simulink model "systemlin"  (R2020b)
settings: Solver=VariableStepAuto  StartTime=0.0  StopTime=10.0  RelTol=1e-3
values from neighbouring files (symbols this model uses):
  a1 = -0.1    [PID_control.m]
  g = p(11,1)    [ModifiedFourTankSystem.m]    (also in approx_MPC_Soft_Output_Input_Constrained.m = [gu;zeros(length(gu),1)]; det_lin_MPC_Soft_Output_Input_Constrained.m = [gu;zeros(length(gu),1)]; noise_nonlin_MPC_Soft_Output_Input_Constrained.m = [gu;zeros(length(gu),1)]; nonlin_MPC_Soft_Output_Input_Constrained.m = [gu;zeros(length(gu),1)])
  rho = p(12,1)    [ModifiedFourTankSystem.m]
undefined symbols (not defined in the file or in its folder): A1, A2, a2, A3, a3, A4, a4, gam1, gam2
settings Model: Creator=maxfi  LastModifiedBy=maxfi

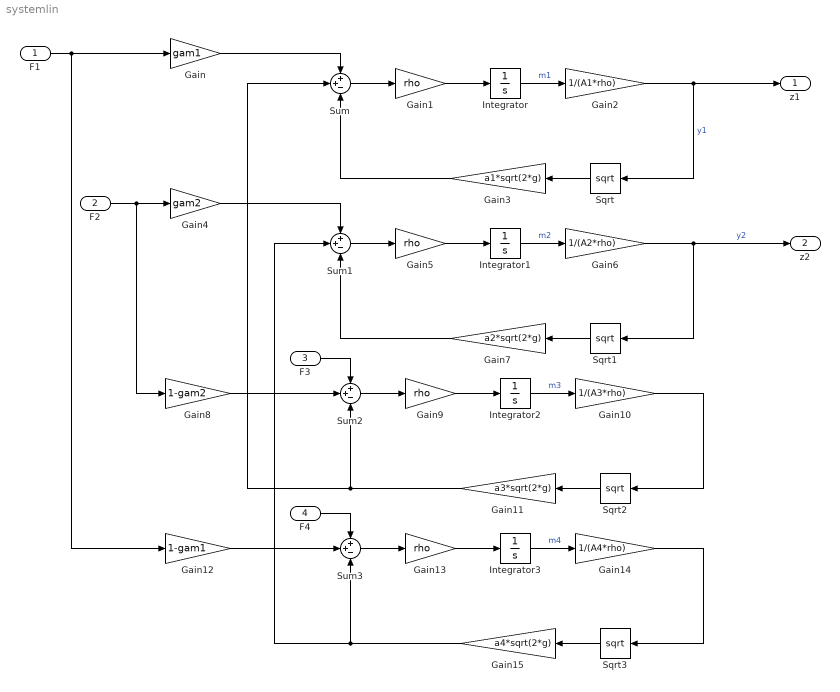
== system systemlin ==
  F1 : Inport
  F2 : Inport  Port=2
  F3 : Inport  Port=3
  F4 : Inport  Port=4
  Gain : Gain  Gain=gam1
  Gain{1,5,9,13} (4 alike) : Gain  Gain=rho
  Gain10 : Gain  Gain=1/(A3*rho)
  Gain11 : Gain  Gain=a3*sqrt(2*g)
  Gain12 : Gain  Gain=1-gam1
  Gain14 : Gain  Gain=1/(A4*rho)
  Gain15 : Gain  Gain=a4*sqrt(2*g)
  Gain2 : Gain  Gain=1/(A1*rho)
  Gain3 : Gain  Gain=a1*sqrt(2*g)
  Gain4 : Gain  Gain=gam2
  Gain6 : Gain  Gain=1/(A2*rho)
  Gain7 : Gain  Gain=a2*sqrt(2*g)
  Gain8 : Gain  Gain=1-gam2
  Integrator : Integrator  Priority=1
  Integrator1 : Integrator  Priority=2
  Integrator2 : Integrator  Priority=3
  Integrator3 : Integrator  Priority=4
  Sqrt{,1..3} (4 alike) : Sqrt  SaturateOnIntegerOverflow=on
  Sum{,1..3} (4 alike) : Sum  Inputs=++-
  z1 : Outport
  z2 : Outport  Port=2
  wires:
  F3/1 -> Sum2/1
  Gain12/1 -> Sum3/2
  Sum/1 -> Gain1/1
  Gain8/1 -> Sum2/2
  Sum1/1 -> Gain5/1
  F4/1 -> Sum3/1
  Gain13/1 -> Integrator3/1
  Gain/1 -> Sum/1
  F1/1 -> Gain12/1, Gain/1
  Sqrt/1 -> Gain3/1
  Sqrt3/1 -> Gain15/1
  Gain15/1 -> Sum1/2, Sum3/3
  Gain5/1 -> Integrator1/1
  Gain14/1 -> Sqrt3/1
  Integrator/1 -> Gain2/1  "m1"
  Gain11/1 -> Sum/2, Sum2/3
  Gain9/1 -> Integrator2/1
  Sqrt2/1 -> Gain11/1
  Gain2/1 -> z1/1, Sqrt/1  "y1"
  Integrator1/1 -> Gain6/1  "m2"
  Gain6/1 -> z2/1, Sqrt1/1  "y2"
  F2/1 -> Gain8/1, Gain4/1
  Gain7/1 -> Sum1/3
  Gain10/1 -> Sqrt2/1
  Integrator3/1 -> Gain14/1  "m4"
  Gain1/1 -> Integrator/1
  Integrator2/1 -> Gain10/1  "m3"
  Sum3/1 -> Gain13/1
  Sqrt1/1 -> Gain7/1
  Sum2/1 -> Gain9/1
  Gain4/1 -> Sum1/1
  Gain3/1 -> Sum/3
